simulink model "DDC_Simulink_v1"  (R2025a)
settings: Solver=VariableStepAuto  StartTime=0.0  StopTime=10.0  RelTol=1e-3
undefined symbols (not defined in the file): h
libraries: dspsrcs4 x1, dsphdlsigops2 x1
settings Model: Creator=icemaster127  LastModifiedBy=icemaster127

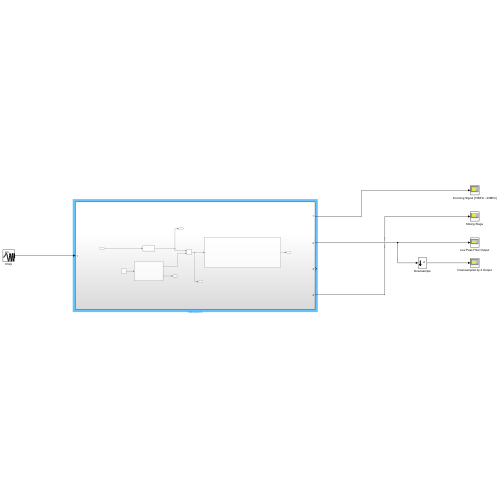
[thumbnail: Simulink's stored preview of the top-level diagram]
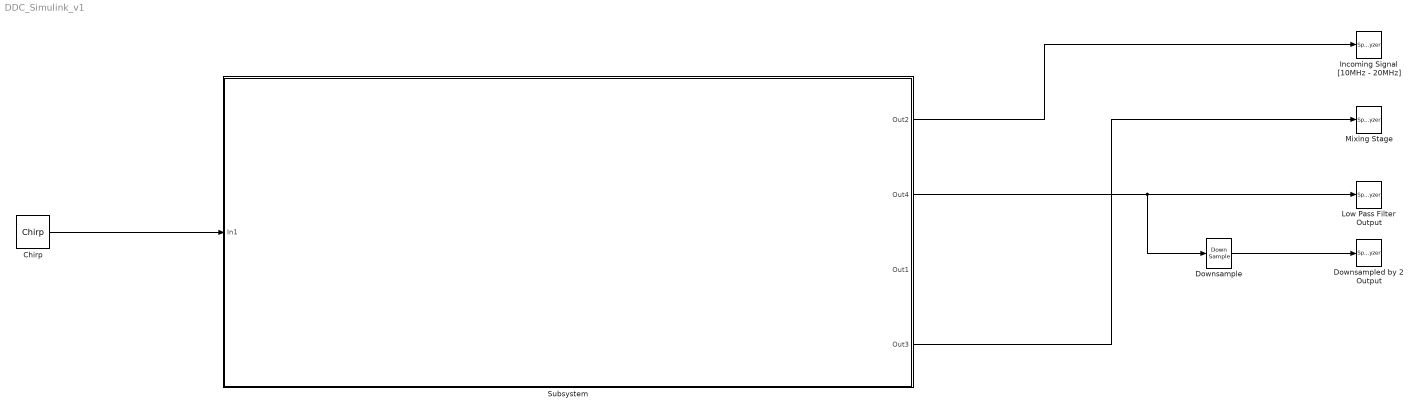
== system DDC_Simulink_v1 ==
  Chirp : dspsrcs4/Chirp  sweep=Linear  mode=Unidirectional  f0=10e6  f1=20e6  t1=.00001998  Tsweep=.00001998  phase=0  Ts=1/1/Fs  spf=1  datatype=double  OutputFrames=off
  Downsample : DownSample  RateOptions=Allow multirate processing
  Downsampled by 2 Output : SpectrumAnalyzer  WindowPosition=[590.000000,545.000000,615.000000,433.000000,]  ScopeFrameLocation=window  WindowInvariantSamplesPerUpdate=on  Span=30000000  StartFrequency=-15000000  StopFrequency=15000000  YLimits=[-45.4477 2.1285]
  Incoming Signal [10MHz - 20MHz] : SpectrumAnalyzer  WindowPosition=[36.000000,124.000000,570.000000,405.000000,]  ScopeFrameLocation=window  WindowInvariantSamplesPerUpdate=on  Span=60000000  StartFrequency=-30000000  StopFrequency=30000000  YLimits=[-41.0011 7.6641]
  Low Pass Filter Output : SpectrumAnalyzer  WindowPosition=[36.000000,557.000000,546.000000,418.000000,]  ScopeFrameLocation=window  WindowInvariantSamplesPerUpdate=on  YLimits=[-163.765 14.5993]
  Mixing Stage : SpectrumAnalyzer  WindowPosition=[614.000000,129.000000,568.000000,411.000000,]  ScopeFrameLocation=window  WindowInvariantSamplesPerUpdate=on  YLimits=[-35.6367 1.1484]
  Subsystem : Subsystem
  wires:
  Chirp/1 -> Subsystem/1(In1)
  Subsystem/1(Out2) -> Incoming Signal [10MHz - 20MHz]/1
  Subsystem/2(Out4) -> Low Pass Filter Output/1, Downsample/1
  Downsample/1 -> Downsampled by 2 Output/1
  Subsystem/4(Out3) -> Mixing Stage/1

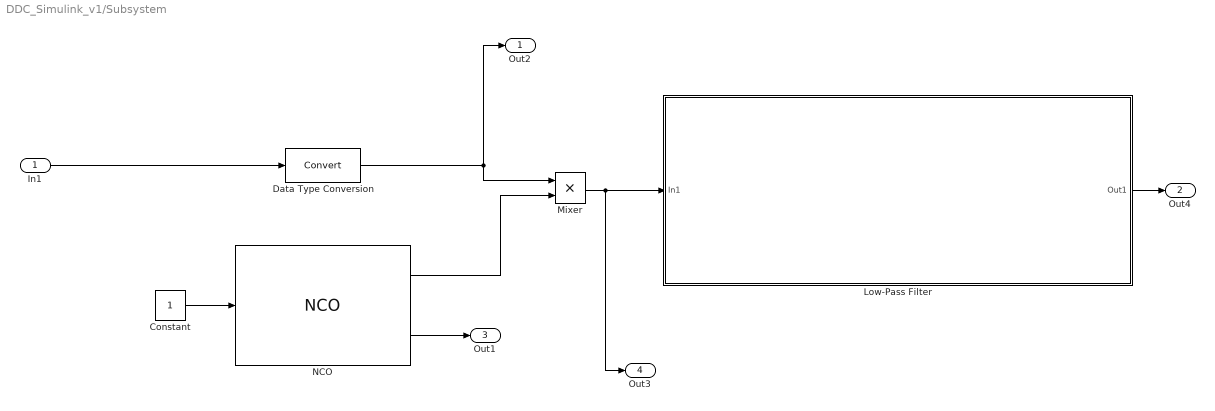
== system DDC_Simulink_v1/Subsystem ==
  In1 : Inport
  Constant : Constant  OutDataTypeStr=boolean
  Data Type Conversion : DataTypeConversion  SaturateOnIntegerOverflow=off  RndMeth=Floor
  Low-Pass Filter : Subsystem
  Mixer : Product
  NCO : dsphdlsigops2/NCO  PhaseIncrementSource=Property  PhaseIncrement=phIncr  PhaseOffsetSource=Property  PhaseOffset=phOff  DitherSource=Property  NumDitherBits=ditherBits  SamplesPerFrame=1  LUTCompress=off  ResetAction=off  Waveform=Cosine  PhasePort=off  SimulateUsing=Code generation  AccumulatorWL=32  PhaseQuantization=on  NumQuantizerAccumulatorBits=12  OutputDataType=Binary point scaling  OutputWL=16  OutputFL=14
      settings: LibrarySourceBlock=dsphdlsrcs2/NCO
  Out2 : Outport
  Out4 : Outport  Port=2
  Out1 : Outport  Port=3
  Out3 : Outport  Port=4
  wires:
  In1/1 -> Data Type Conversion/1
  Data Type Conversion/1 -> Out2/1, Mixer/1
  NCO/1 -> Mixer/2
  NCO/2 -> Out1/1
  Mixer/1 -> Out3/1, Low-Pass Filter/1(In1)
  Low-Pass Filter/1(Out1) -> Out4/1
  Constant/1 -> NCO/1

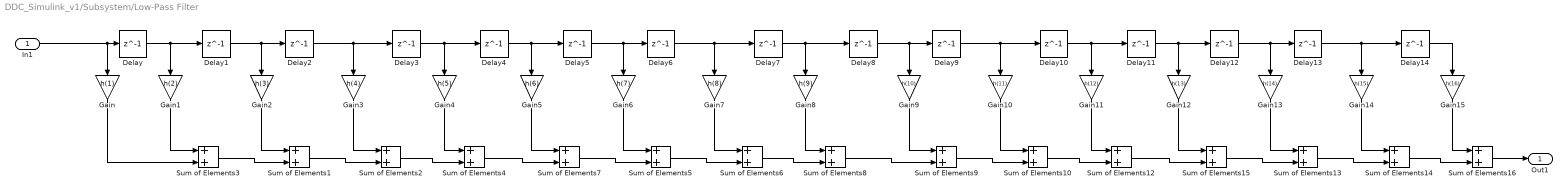
== system DDC_Simulink_v1/Subsystem/Low-Pass Filter ==
  In1 : Inport
  Delay{,1..14} (15 alike) : Delay  DelayLength=1
  Gain : Gain  Gain=h(1)
  Gain1 : Gain  Gain=h(2)
  Gain10 : Gain  Gain=h(11)
  Gain11 : Gain  Gain=h(12)
  Gain12 : Gain  Gain=h(13)
  Gain13 : Gain  Gain=h(14)
  Gain14 : Gain  Gain=h(15)
  Gain15 : Gain  Gain=h(16)
  Gain2 : Gain  Gain=h(3)
  Gain3 : Gain  Gain=h(4)
  Gain4 : Gain  Gain=h(5)
  Gain5 : Gain  Gain=h(6)
  Gain6 : Gain  Gain=h(7)
  Gain7 : Gain  Gain=h(8)
  Gain8 : Gain  Gain=h(9)
  Gain9 : Gain  Gain=h(10)
  Sum of Elements{1..10,12..16} (15 alike) : Sum
  Out1 : Outport
  wires:
  Delay1/1 -> Delay2/1, Gain2/1
  Delay/1 -> Delay1/1, Gain1/1
  In1/1 -> Gain/1, Delay/1
  Delay3/1 -> Delay4/1, Gain4/1
  Gain3/1 -> Sum of Elements2/1
  Delay2/1 -> Delay3/1, Gain3/1
  Sum of Elements1/1 -> Sum of Elements2/2
  Gain2/1 -> Sum of Elements1/1
  Sum of Elements3/1 -> Sum of Elements1/2
  Gain1/1 -> Sum of Elements3/1
  Gain/1 -> Sum of Elements3/2
  Gain4/1 -> Sum of Elements4/1
  Sum of Elements2/1 -> Sum of Elements4/2
  Sum of Elements5/1 -> Sum of Elements6/2
  Gain8/1 -> Sum of Elements8/1
  Delay6/1 -> Delay7/1, Gain7/1
  Delay4/1 -> Delay5/1, Gain5/1
  Delay5/1 -> Delay6/1, Gain6/1
  Delay7/1 -> Delay8/1, Gain8/1
  Sum of Elements7/1 -> Sum of Elements5/2
  Gain7/1 -> Sum of Elements6/1
  Gain5/1 -> Sum of Elements7/1
  Sum of Elements6/1 -> Sum of Elements8/2
  Gain6/1 -> Sum of Elements5/1
  Sum of Elements4/1 -> Sum of Elements7/2
  Gain14/1 -> Sum of Elements14/1
  Gain13/1 -> Sum of Elements13/1
  Sum of Elements9/1 -> Sum of Elements10/2
  Gain11/1 -> Sum of Elements12/1
  Gain12/1 -> Sum of Elements15/1
  Delay12/1 -> Delay13/1, Gain13/1
  Sum of Elements14/1 -> Sum of Elements16/2
  Delay11/1 -> Delay12/1, Gain12/1
  Gain15/1 -> Sum of Elements16/1
  Delay13/1 -> Delay14/1, Gain14/1
  Sum of Elements13/1 -> Sum of Elements14/2
  Delay9/1 -> Delay10/1, Gain10/1
  Delay8/1 -> Delay9/1, Gain9/1
  Gain10/1 -> Sum of Elements10/1
  Sum of Elements10/1 -> Sum of Elements12/2
  Sum of Elements12/1 -> Sum of Elements15/2
  Delay10/1 -> Delay11/1, Gain11/1
  Sum of Elements15/1 -> Sum of Elements13/2
  Gain9/1 -> Sum of Elements9/1
  Delay14/1 -> Gain15/1
  Sum of Elements8/1 -> Sum of Elements9/2
  Sum of Elements16/1 -> Out1/1
